simulink model "testWriteActiveMQ_cpp"  (R2018b)
settings: Solver=FixedStepDiscrete  StartTime=0.0  StopTime=inf  FixedStep=0.001  RelTol=1e-3  EnableMultiTasking=on
model workspace (MAT data in the model file):
  gtest = 0
libraries: activeMQ x2, VCTlbx x2
settings Model: Creator=Ulysses  LastModifiedBy=Ulysses
settings DataIOCC: LimitDataPoints=on  SaveFormat=Array
settings OptimizationCC: LifeSpan=inf
settings DebuggingCC: SolverPrmCheckMsg=warning  AllowSymbolicDim=off  SFUnexpectedBacktrackingDiag=warning  SFNoUnconditionalDefaultTransitionDiag=warning
settings HardwareCC: ProdBitPerPointer=32  ProdBitPerSizeT=32  ProdBitPerPtrDiffT=32  ProdLargestAtomicFloat=None  ProdIntDivRoundTo=Undefined  ProdEndianess=Unspecified  ProdWordSize=32  ProdHWDeviceType=32-bit Generic
settings ModelReferenceCC: PropagateSignalLabelsOutOfModel=off
settings SFSimCC: SimUseLocalCustomCode=off
settings RTWCC: RTWUseLocalCustomCode=off  TargetLang=C++
settings CodeAppCC: StateflowObjectComments=on
settings GRTTargetCC: TargetLangStandard=C89/C90 (ANSI)  GeneratePreprocessorConditionals=Disable all  MultiInstanceERTCode=on  CodeInterfacePackaging=C++ class
settings ConfigComp: CovMetricSettings=dw  CovHtmlReporting=on  CovSaveCumulativeToWorkspaceVar=on  CovSaveSingleToWorkspaceVar=on  CovExternalEMLEnable=off  CovSFcnEnable=off

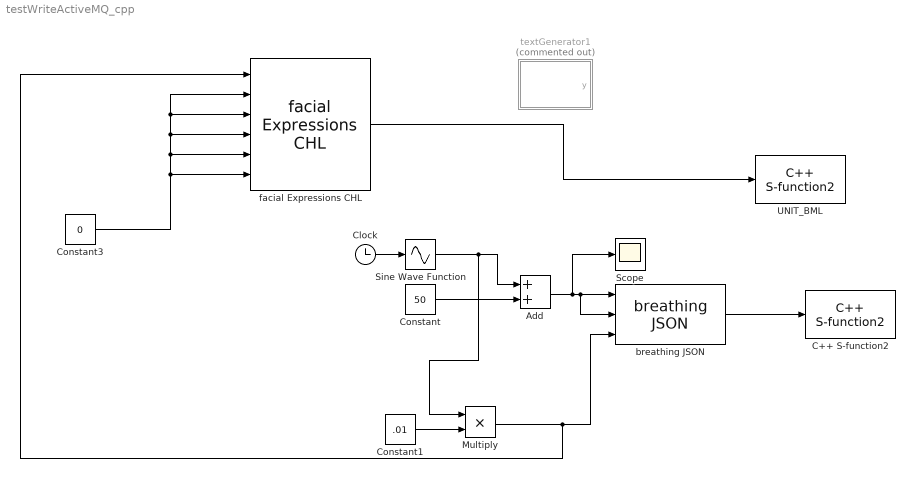
== system testWriteActiveMQ_cpp ==
  Add : Sum
  C++ S-function2 : activeMQ/C++ S-function2  server='127.0.0.1'  port='61616'  scope=UNITY_JSON  character='FuseCharacter'
      settings: SourceProductName=activeMQ
  Clock : Clock
  Constant : Constant  Value=50
  Constant1 : Constant  Value=.01
  Constant3 : Constant  Value=0
  Multiply : Product
  Scope : Scope
  Sine Wave Function : Sin  TimeSource=Use external signal  Amplitude=50  Frequency=50  SampleTime=0
  "UNIT_BML " : activeMQ/C++ S-function2  server='localhost'  port='61616'  scope=UNITY_BML  character='FuseCharacter'
      settings: SourceProductName=activeMQ
  breathing JSON : VCTlbx/breathing JSON  charname='FuseCharacter'
      settings: SourceProductName=Virtual Character Toolbox
  facial Expressions CHL : VCTlbx/facial Expressions CHL
      settings: SourceProductName=Virtual Character Toolbox
  textGenerator1 : MATLAB Function  Commented=on  TreatAsAtomicUnit=on
  wires:
  facial Expressions CHL/1 -> "UNIT_BML "/1
  breathing JSON/1 -> C++ S-function2/1
  Sine Wave Function/1 -> Multiply/1, Add/1
  Clock/1 -> Sine Wave Function/1
  Constant/1 -> Add/2
  Add/1 -> breathing JSON/2, breathing JSON/1, Scope/1
  Multiply/1 -> facial Expressions CHL/1, breathing JSON/3
  Constant1/1 -> Multiply/2
  Constant3/1 -> facial Expressions CHL/6, facial Expressions CHL/5, facial Expressions CHL/4, facial Expressions CHL/3, facial Expressions CHL/2

== matlab function testWriteActiveMQ_cpp/textGenerator1 ==
  data: y output
function y = fcn()
y = encStr2Arr('<?xml version="1.0" ?><act><bml><face au="12" side="BOTH" type="facs" amount="1"/></bml></act>');
